simulink library "reelOut"  (R2018a)
settings: Solver=VariableStepAuto  StartTime=0.0  StopTime=10.0  RelTol=1e-3
undefined symbols (not defined in the file or in its folder): ctrl
libraries: controllerComponents x6, simulink x2
settings Model: Creator=mitch  LastModifiedBy=mitch

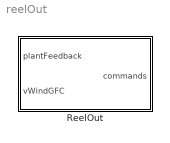
== system reelOut ==
  ReelOut : Subsystem  VariantControl=variantOCK

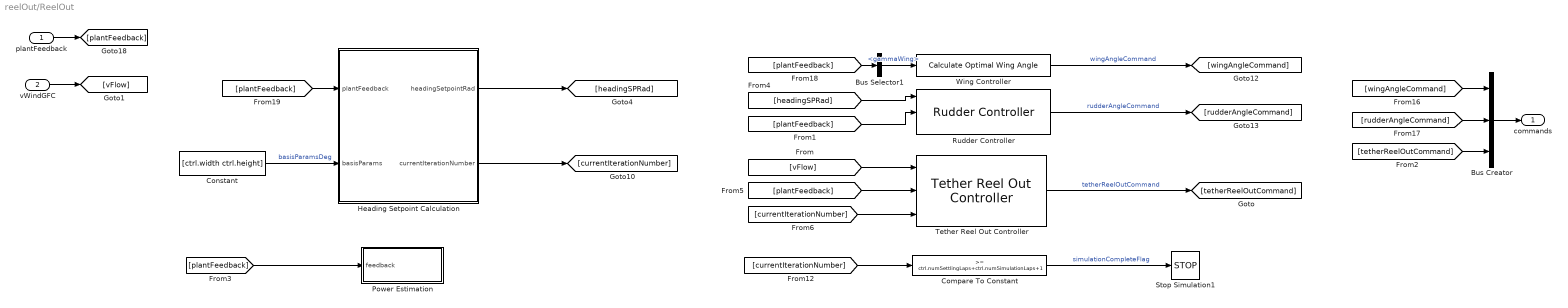
== system reelOut/ReelOut ==
  plantFeedback : Inport  OutDataTypeStr=Bus: busPlantFeedback
  vWindGFC : Inport  Port=2
  Bus Creator : BusCreator  Inputs=3  OutDataTypeStr=Bus: busControllerOutput
  Bus Selector1 : BusSelector  OutputSignals=gammaWing
  Compare To Constant : simulink/Logic and Bit Operations/Compare To Constant  relop=>=  const=ctrl.numSettlingLaps+ctrl.numSimulationLaps+1  OutDataTypeStr=boolean
  Constant : Constant  Value=[ctrl.width ctrl.height]
  Heading Setpoint Calculation : Subsystem  VariantControl=variantPureCarrotFollowing
  Power Estimation : Subsystem
  Rudder Controller : controllerComponents/Rudder Controller
  Stop Simulation1 : Stop
  Tether Reel Out Controller : controllerComponents/Tether Reel Out Controller
  Wing Controller : controllerComponents/Calculate Optimal Wing Angle
  commands : Outport  OutDataTypeStr=Bus: busControllerOutput
  wires:
  [currentIterationNumber] -> Tether Reel Out Controller/3
  [plantFeedback] -> Tether Reel Out Controller/2
  [plantFeedback] -> Power Estimation/1(feedback)
  [vFlow] -> Tether Reel Out Controller/1
  Tether Reel Out Controller/1 -> [tetherReelOutCommand]  "tetherReelOutCommand"
  [tetherReelOutCommand] -> Bus Creator/3
  Wing Controller/1 -> [wingAngleCommand]  "wingAngleCommand"
  Rudder Controller/1 -> [rudderAngleCommand]  "rudderAngleCommand"
  [headingSPRad] -> Rudder Controller/1
  Heading Setpoint Calculation/1(headingSetpointRad) -> [headingSPRad]
  Heading Setpoint Calculation/2(currentIterationNumber) -> [currentIterationNumber]
  Compare To Constant/1 -> Stop Simulation1/1  "simulationCompleteFlag"
  [currentIterationNumber] -> Compare To Constant/1
  [wingAngleCommand] -> Bus Creator/1
  [rudderAngleCommand] -> Bus Creator/2
  Bus Creator/1 -> commands/1
  Bus Selector1/1 -> Wing Controller/1  "<gammaWing>"
  vWindGFC/1 -> [vFlow]
  plantFeedback/1 -> [plantFeedback]
  [plantFeedback] -> Bus Selector1/1
  [plantFeedback] -> Rudder Controller/2
  Constant/1 -> Heading Setpoint Calculation/2(basisParams)  "basisParamsDeg"
  [plantFeedback] -> Heading Setpoint Calculation/1(plantFeedback)

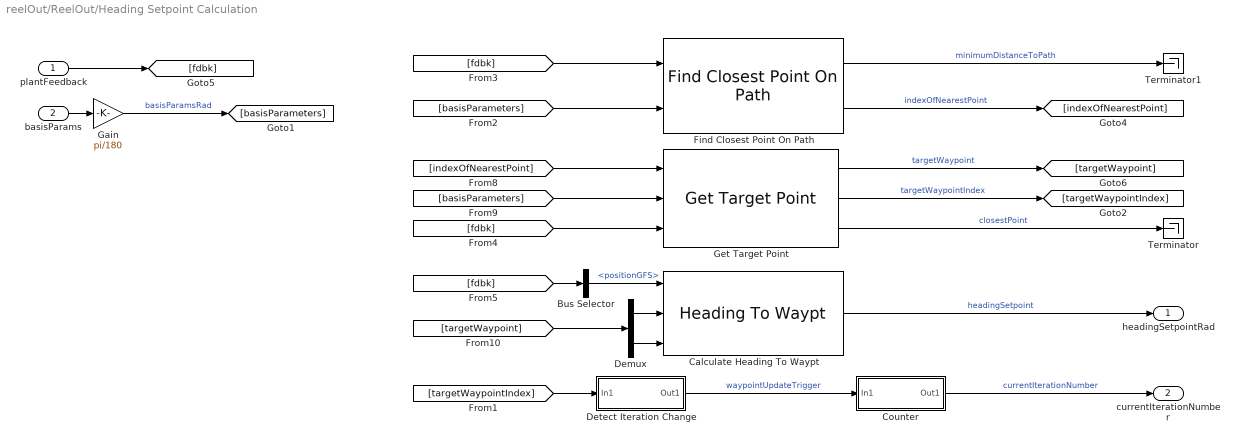
== system reelOut/ReelOut/Heading Setpoint Calculation ==
  plantFeedback : Inport  OutDataTypeStr=Bus: busPlantFeedback
  basisParams : Inport  Port=2
  Bus Selector : BusSelector  OutputSignals=positionGFS
  Calculate Heading To Waypt : controllerComponents/Heading To Waypt
  Counter : Subsystem
  Demux : Demux  Outputs=2
  Detect Iteration Change : Subsystem
  Find Closest Point On Path : controllerComponents/Find Closest Point On Path
  Gain : Gain  Gain=pi/180
  Get Target Point : controllerComponents/Get Target Point
  Terminator : Terminator
  Terminator1 : Terminator
  headingSetpointRad : Outport
  currentIterationNumber : Outport  Port=2
  wires:
  Gain/1 -> [basisParameters]  "basisParamsRad"
  Bus Selector/1 -> Calculate Heading To Waypt/1  "<positionGFS>"
  [fdbk] -> Bus Selector/1
  basisParams/1 -> Gain/1
  [fdbk] -> Get Target Point/3
  [fdbk] -> Find Closest Point On Path/1
  [basisParameters] -> Find Closest Point On Path/2
  Demux/1 -> Calculate Heading To Waypt/2
  Demux/2 -> Calculate Heading To Waypt/3
  Find Closest Point On Path/1 -> Terminator1/1  "minimumDistanceToPath"
  Find Closest Point On Path/2 -> [indexOfNearestPoint]  "indexOfNearestPoint"
  [indexOfNearestPoint] -> Get Target Point/1
  [basisParameters] -> Get Target Point/2
  Get Target Point/1 -> [targetWaypoint]  "targetWaypoint"
  [targetWaypoint] -> Demux/1
  Calculate Heading To Waypt/1 -> headingSetpointRad/1  "headingSetpoint"
  [targetWaypointIndex] -> Detect Iteration Change/1(In1)
  Counter/1(Out1) -> currentIterationNumber/1  "currentIterationNumber"
  Detect Iteration Change/1(Out1) -> Counter/1(In1)  "waypointUpdateTrigger"
  Get Target Point/2 -> [targetWaypointIndex]  "targetWaypointIndex"
  plantFeedback/1 -> [fdbk]
  Get Target Point/3 -> Terminator/1  "closestPoint"

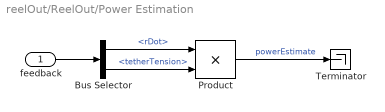
== system reelOut/ReelOut/Power Estimation ==
  feedback : Inport
  Bus Selector : BusSelector  OutputSignals=rDot,tetherTension
  Product : Product
  Terminator : Terminator
  wires:
  Bus Selector/2 -> Product/2  "<tetherTension>"
  Bus Selector/1 -> Product/1  "<rDot>"
  feedback/1 -> Bus Selector/1
  Product/1 -> Terminator/1  "powerEstimate"

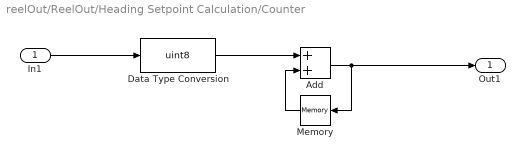
== system reelOut/ReelOut/Heading Setpoint Calculation/Counter ==
  In1 : Inport
  Add : Sum
  Data Type Conversion : DataTypeConversion  OutDataTypeStr=uint8
  Memory : Memory  InitialCondition=1
  Out1 : Outport  OutDataTypeStr=double
  wires:
  Add/1 -> Out1/1, Memory/1
  Memory/1 -> Add/2
  In1/1 -> Data Type Conversion/1
  Data Type Conversion/1 -> Add/1

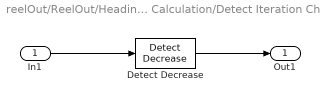
== system reelOut/ReelOut/Heading Setpoint Calculation/Detect Iteration Change ==
  In1 : Inport
  Detect Decrease : simulink/Logic and Bit Operations/Detect Decrease  vinit=0.0  OutDataTypeStr=boolean
  Out1 : Outport
  wires:
  In1/1 -> Detect Decrease/1
  Detect Decrease/1 -> Out1/1
